simulink model "PF_Simulink_TEST"  (R2022b)
settings: Solver=FixedStepAuto  StartTime=0.0  StopTime=25  FixedStep=0.10  RelTol=1e-3
values from neighbouring files (symbols this model uses):
  D1 = W2_newnew(x0)    [main_S_F.m]
  D2 = W3_newnew(x0)    [main_S_F.m]
  num_particles = 75    [main_S_F.m]
  std_dev1 = std_dev    [main_S_F.m]
  std_dev2 = [1.5; 1.5; 1e-3; 1e-3; 1e-6; 0.2;0.2]    [main_S_F.m]
  W_xu_ranges = [ ... (first row only)    [main_S_F.m]
  W_xucar1 = [10;10;1e-4;1e-4;1e-4;0.50;0.1]    [main_S_F.m]
  W_xucar2 = [10;10;1e-4;1e-4;1e-4;0.50;0.1]    [main_S_F.m]
  x0 = [0;-45;pi/2;0;0;-30;0;0;10;0]    [main_S_F.m]
undefined symbols (not defined in the file or in its folder): estimated_W_xu_car2, estimated_Wxu_car1
(part 1 of 2)
settings Model: PauseTimes=10  Creator=user  LastModifiedBy=user

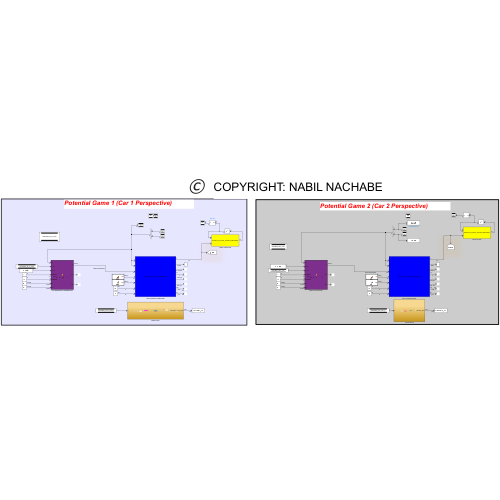
[thumbnail: Simulink's stored preview of the top-level diagram]
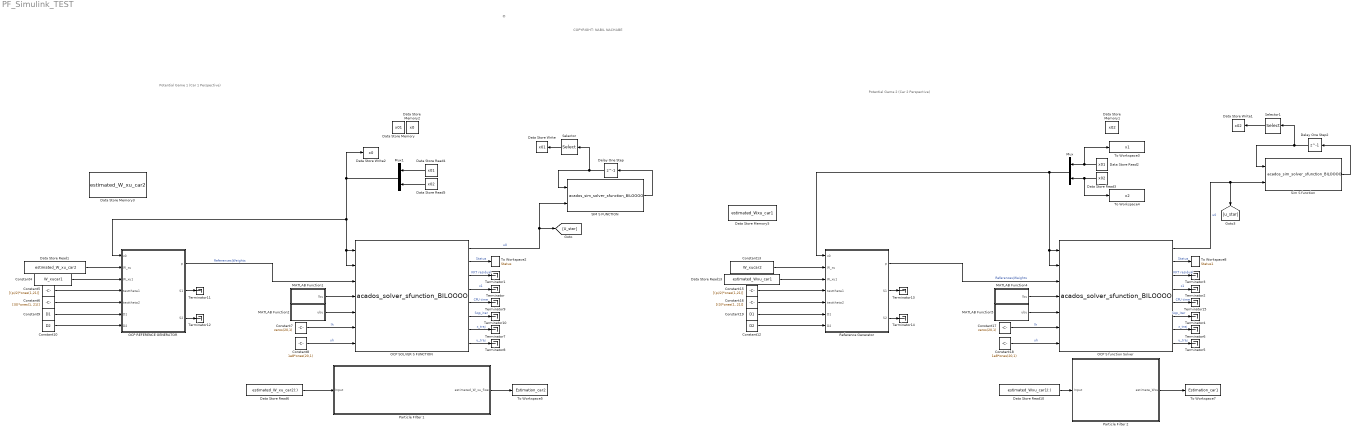
== system PF_Simulink_TEST ==
  note: ©
  note: COPYRIGHT: NABIL NACHABE
  note: Potential Game 2 (Car 2 Perspective)
  note: Potential Game 1 (Car 1 Perspective)
  Constant10 : Constant  Value=D2
  Constant12 : Constant  Value=D2
  Constant13 : Constant  Value=W_xucar2
  Constant15 : Constant  Value=[(pi/2)*ones(1,21)]
  Constant16 : Constant  Value=[(0)*ones(1, 21)]
  Constant17 : Constant  Value=zeros(20,1)
  Constant18 : Constant  Value=1e8*ones(20,1)
  Constant19 : Constant  Value=D1
  Constant4 : Constant  Value=W_xucar1
  Constant5 : Constant  Value=[(pi/2)*ones(1,21)]
  Constant6 : Constant  Value=[(0)*ones(1, 21)]
  Constant7 : Constant  Value=zeros(20,1)
  Constant8 : Constant  Value=1e8*ones(20,1)
  Constant9 : Constant  Value=D1
  Data Store Memory : DataStoreMemory  DataStoreName=x01  WriteAfterWriteMsg=warning  InitialValue=x01  ShowAdditionalParam=off
  Data Store Memory1 : DataStoreMemory  DataStoreName=x02  WriteAfterWriteMsg=warning  InitialValue=x02  ShowAdditionalParam=off
  Data Store Memory2 : DataStoreMemory  DataStoreName=x0  WriteAfterWriteMsg=warning  InitialValue=x0  ShareAcrossModelInstances=on  ShowAdditionalParam=off
  Data Store Memory3 : DataStoreMemory  DataStoreName=estimated_W_xu_car2  WriteAfterWriteMsg=warning  InitialValue=initial_guess_belief_car2  ShowAdditionalParam=off
  Data Store Memory5 : DataStoreMemory  DataStoreName=estimated_Wxu_car1  WriteAfterWriteMsg=warning  InitialValue=initial_guess_belief_car1  ShowAdditionalParam=off
  Data Store Read1 : DataStoreRead  DataStoreName=estimated_W_xu_car2  IndexOptions=Index vector (dialog)  Indices=1  OutputSizes=1
  Data Store Read10 : DataStoreRead  DataStoreName=estimated_Wxu_car1  DataStoreElements=estimated_Wxu_car1(:)  IndexOptions=Index vector (dialog)  Indices=1  OutputSizes=1
  Data Store Read13 : DataStoreRead  DataStoreName=estimated_Wxu_car1  IndexOptions=Index vector (dialog)  Indices=1  OutputSizes=1
  Data Store Read2 : DataStoreRead  DataStoreName=x01  IndexOptions=Index vector (dialog)  Indices=1  OutputSizes=1
  Data Store Read3 : DataStoreRead  DataStoreName=x02  IndexOptions=Index vector (dialog)  Indices=1  OutputSizes=1
  Data Store Read4 : DataStoreRead  DataStoreName=x01  IndexOptions=Index vector (dialog)  Indices=1  OutputSizes=1
  Data Store Read5 : DataStoreRead  DataStoreName=x02  IndexOptions=Index vector (dialog)  Indices=1  OutputSizes=1
  Data Store Read6 : DataStoreRead  DataStoreName=estimated_W_xu_car2  DataStoreElements=estimated_W_xu_car2(:)  IndexOptions=Index vector (dialog)  Indices=1  OutputSizes=1
  Data Store Write : DataStoreWrite  DataStoreName=x01  DataStoreElements=x01  IndexOptions=Index vector (dialog)  Indices=1  OutputSizes=1
  Data Store Write1 : DataStoreWrite  DataStoreName=x02  IndexOptions=Index vector (dialog)  Indices=1  OutputSizes=1
  Data Store Write2 : DataStoreWrite  DataStoreName=x0  IndexOptions=Index vector (dialog)  Indices=1  OutputSizes=1
  Delay One Step : Delay  DelayLength=1  InitialCondition=x0
  Delay One Step2 : Delay  DelayLength=1  InitialCondition=x0
  MATLAB Function1 : MATLAB Function  TreatAsAtomicUnit=on
  MATLAB Function2 : MATLAB Function  TreatAsAtomicUnit=on
  MATLAB Function4 : MATLAB Function  TreatAsAtomicUnit=on
  MATLAB Function5 : MATLAB Function  TreatAsAtomicUnit=on
  Mux : Mux  Inputs=2
  Mux1 : Mux  Inputs=2
  OCP REFERENCE GENERATOR : MATLAB Function  TreatAsAtomicUnit=on
  OCP S function Solver : S-Function  FunctionName=acados_solver_sfunction_BILOOOO  SFunctionDeploymentMode=off  EnableBusSupport=off
  OCP SOLVER S FUNCTION : S-Function  FunctionName=acados_solver_sfunction_BILOOOO  SFunctionDeploymentMode=off  EnableBusSupport=off
  Particle FIlter 1 : Subsystem
  Particle Filter 2 : Subsystem
  Reference Generator : MATLAB Function  TreatAsAtomicUnit=on
  SIM S FUNCTION : S-Function  FunctionName=acados_sim_solver_sfunction_BILOOOO  SFunctionDeploymentMode=off  EnableBusSupport=off
  Selector : Selector  InputPortWidth=10  IndexOptions=Index vector (dialog)  Indices=[1:5]  OutputSizes=1
  Selector1 : Selector  InputPortWidth=10  IndexOptions=Index vector (dialog)  Indices=[6:10]  OutputSizes=1
  Sim S function : S-Function  FunctionName=acados_sim_solver_sfunction_BILOOOO  SFunctionDeploymentMode=off  EnableBusSupport=off
  Terminator{,1..15} (16 alike) : Terminator
  To Workspace2 : ToWorkspace  VariableName=Status  SampleTime=-1
      settings: Save2DSignal=2-D array (concatenate along first dimension)
  To Workspace3 : ToWorkspace  VariableName=x1  SaveFormat=Structure  SampleTime=-1
  To Workspace4 : ToWorkspace  VariableName=x2  SaveFormat=Structure  SampleTime=-1
  To Workspace5 : ToWorkspace  VariableName=Estimation_car2  SampleTime=-1
      settings: Save2DSignal=2-D array (concatenate along first dimension)
  To Workspace7 : ToWorkspace  VariableName=Estimation_car1  SampleTime=-1
      settings: Save2DSignal=2-D array (concatenate along first dimension)
  To Workspace8 : ToWorkspace  VariableName=Status1  SampleTime=-1
      settings: Save2DSignal=2-D array (concatenate along first dimension)
  wires:
  Data Store Read13/1 -> Reference Generator/3(W_xu1)
  Mux1/1 -> Data Store Write2/1, OCP SOLVER S FUNCTION/2, OCP SOLVER S FUNCTION/1, OCP REFERENCE GENERATOR/1(x0)
  Data Store Read5/1 -> Mux1/2
  Sim S function/1 -> Delay One Step2/1
  Constant19/1 -> Reference Generator/6(D1)
  Constant15/1 -> Reference Generator/4(testtheta1)
  Constant7/1 -> OCP SOLVER S FUNCTION/6  "lh"
  MATLAB Function1/1(lbu) -> OCP SOLVER S FUNCTION/4
  OCP REFERENCE GENERATOR/2(S1) -> Terminator11/1
  OCP REFERENCE GENERATOR/1(p) -> OCP SOLVER S FUNCTION/3  "References|Weights"
  OCP SOLVER S FUNCTION/4 -> Terminator/1  "x1"
  Data Store Read3/1 -> To Workspace4/1, Mux/2
  Reference Generator/3(S2) -> Terminator14/1
  OCP S function Solver/7 -> Terminator6/1  "x_traj"
  OCP SOLVER S FUNCTION/3 -> Terminator1/1  "KKT residual"
  MATLAB Function4/1(lbu) -> OCP S function Solver/4
  Delay One Step/1 -> Selector/1, SIM S FUNCTION/1
  Constant13/1 -> Reference Generator/2(W_xu)
  Constant17/1 -> OCP S function Solver/6  "lh"
  SIM S FUNCTION/1 -> Delay One Step/1
  Constant8/1 -> OCP SOLVER S FUNCTION/7  "uh"
  OCP REFERENCE GENERATOR/3(S2) -> Terminator12/1
  Delay One Step2/1 -> Selector1/1, Sim S function/1
  OCP SOLVER S FUNCTION/2 -> To Workspace2/1  "Status"
  OCP S function Solver/2 -> To Workspace8/1  "Status"
  Reference Generator/1(p) -> OCP S function Solver/3  "References|Weights"
  MATLAB Function5/1(ubu) -> OCP S function Solver/5
  OCP S function Solver/3 -> Terminator3/1  "KKT residual"
  Constant10/1 -> OCP REFERENCE GENERATOR/7(D2)
  OCP SOLVER S FUNCTION/8 -> Terminator8/1  "u_traj"
  OCP S function Solver/5 -> Terminator15/1  "CPU time"
  OCP S function Solver/4 -> Terminator2/1  "x1"
  Constant4/1 -> OCP REFERENCE GENERATOR/3(W_xu1)
  Constant16/1 -> Reference Generator/5(testtheta2)
  MATLAB Function2/1(ubu) -> OCP SOLVER S FUNCTION/5
  Mux/1 -> OCP S function Solver/2, OCP S function Solver/1, Reference Generator/1(x0)
  Data Store Read4/1 -> Mux1/1
  OCP S function Solver/6 -> Terminator4/1  "Sqp_iter"
  Constant6/1 -> OCP REFERENCE GENERATOR/5(testtheta2)
  OCP S function Solver/1 -> Sim S function/2, [u_star]  "u0"
  OCP SOLVER S FUNCTION/6 -> Terminator10/1  "Sqp_iter"
  OCP SOLVER S FUNCTION/1 -> SIM S FUNCTION/2, [U_star]  "u0"
  Reference Generator/2(S1) -> Terminator13/1
  OCP S function Solver/8 -> Terminator5/1  "u_traj"
  Constant5/1 -> OCP REFERENCE GENERATOR/4(testtheta1)
  Selector/1 -> Data Store Write/1
  Selector1/1 -> Data Store Write1/1
  OCP SOLVER S FUNCTION/5 -> Terminator9/1  "CPU time"
  Constant9/1 -> OCP REFERENCE GENERATOR/6(D1)
  OCP SOLVER S FUNCTION/7 -> Terminator7/1  "x_traj"
  Data Store Read2/1 -> To Workspace3/1, Mux/1
  Constant12/1 -> Reference Generator/7(D2)
  Constant18/1 -> OCP S function Solver/7  "uh"
  Data Store Read1/1 -> OCP REFERENCE GENERATOR/2(W_xu)
  Data Store Read6/1 -> Particle FIlter 1/1(Input)
  Particle FIlter 1/1(estimated_W_xu_fixed) -> To Workspace5/1
  Data Store Read10/1 -> Particle Filter 2/1(Input)
  Particle Filter 2/1(estimate_Wxu) -> To Workspace7/1

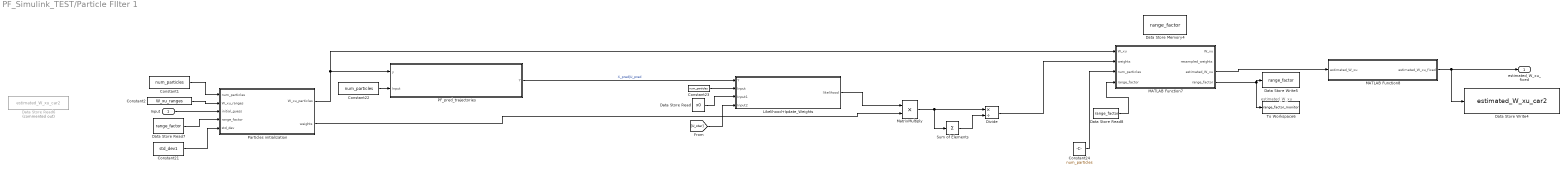
== system PF_Simulink_TEST/Particle FIlter 1 ==
  note: estimated_W_xu
  Input : Inport
  Constant{1,22..24} (4 alike) : Constant  Value=num_particles
  Constant2 : Constant  Value=W_xu_ranges
  Constant21 : Constant  Value=std_dev1
  Data Store Memory4 : DataStoreMemory  DataStoreName=range_factor  WriteAfterWriteMsg=warning  InitialValue=1  ShowAdditionalParam=off
  Data Store Read : DataStoreRead  DataStoreName=x0  IndexOptions=Index vector (dialog)  Indices=1  OutputSizes=1
  Data Store Read6 : DataStoreRead  Commented=on  DataStoreName=estimated_W_xu_car2  IndexOptions=Index vector (dialog)  Indices=1  OutputSizes=1
  Data Store Read7 : DataStoreRead  DataStoreName=range_factor  IndexOptions=Index vector (dialog)  Indices=1  OutputSizes=1
  Data Store Read8 : DataStoreRead  DataStoreName=range_factor  IndexOptions=Index vector (dialog)  Indices=1  OutputSizes=1
  Data Store Write4 : DataStoreWrite  DataStoreName=estimated_W_xu_car2  IndexOptions=Index vector (dialog)  Indices=1  OutputSizes=1
  Data Store Write5 : DataStoreWrite  DataStoreName=range_factor  IndexOptions=Index vector (dialog)  Indices=1  OutputSizes=1
  Divide : Product  Inputs=*/
  Likelihood+Ipdate_Weights : Subsystem  TreatAsAtomicUnit=on
  MATLAB Function7 : MATLAB Function  TreatAsAtomicUnit=on
  MATLAB Function8 : MATLAB Function  TreatAsAtomicUnit=on
  MatrixMultiply : Product
  PF_pred_trajectories : Subsystem  TreatAsAtomicUnit=on
  Particles initialization : MATLAB Function  TreatAsAtomicUnit=on
  Sum of Elements : Sum  Inputs=+
  To Workspace6 : ToWorkspace  VariableName=range_factor_monitor  SampleTime=-1
      settings: Save2DSignal=2-D array (concatenate along first dimension)
  estimated_W_xu_fixed : Outport
  wires:
  Data Store Read7/1 -> Particles initialization/4(range_factor)
  Constant1/1 -> Particles initialization/1(num_particles)
  MATLAB Function8/1(estimated_W_xu_fixed) -> Data Store Write4/1, estimated_W_xu_fixed/1
  Constant23/1 -> Likelihood+Ipdate_Weights/2(Input)
  Particles initialization/1(W_xu_particles) -> MATLAB Function7/1("W_xu "), PF_pred_trajectories/1(y)
  Constant22/1 -> PF_pred_trajectories/2(Input)
  PF_pred_trajectories/1(Y) -> Likelihood+Ipdate_Weights/1(Y)  "X_pred|U_pred"
  Likelihood+Ipdate_Weights/1(likelihood) -> MatrixMultiply/1
  Sum of Elements/1 -> Divide/2
  Particles initialization/2(weights) -> MatrixMultiply/2
  Data Store Read/1 -> Likelihood+Ipdate_Weights/3(Input1)
  Constant24/1 -> MATLAB Function7/3(num_particles)
  MatrixMultiply/1 -> Sum of Elements/1, Divide/1
  Data Store Read8/1 -> MATLAB Function7/4("range_factor ")
  MATLAB Function7/4(range_factor) -> Data Store Write5/1, To Workspace6/1
  MATLAB Function7/3(estimated_W_xu) -> MATLAB Function8/1(estimated_W_xu)
  [U_star] -> Likelihood+Ipdate_Weights/4(Input2)
  Constant2/1 -> Particles initialization/2(W_xu_ranges)
  Divide/1 -> MATLAB Function7/2(weights)
  Input/1 -> Particles initialization/3(initial_guess)
  Constant21/1 -> Particles initialization/5(std_dev)

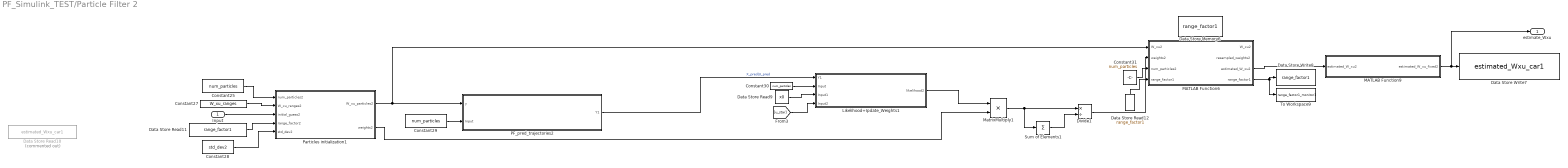
== system PF_Simulink_TEST/Particle Filter 2 ==
  Input : Inport
  Constant{25,29..31} (4 alike) : Constant  Value=num_particles
  Constant27 : Constant  Value=W_xu_ranges
  Constant28 : Constant  Value=std_dev2
  Data Store Memory6 : DataStoreMemory  DataStoreName=range_factor1  WriteAfterWriteMsg=warning  InitialValue=1  ShowAdditionalParam=off
  Data Store Read10 : DataStoreRead  Commented=on  DataStoreName=estimated_Wxu_car1  IndexOptions=Index vector (dialog)  Indices=1  OutputSizes=1
  Data Store Read11 : DataStoreRead  DataStoreName=range_factor1  IndexOptions=Index vector (dialog)  Indices=1  OutputSizes=1
  Data Store Read12 : DataStoreRead  DataStoreName=range_factor1  IndexOptions=Index vector (dialog)  Indices=1  OutputSizes=1
  Data Store Read9 : DataStoreRead  DataStoreName=x0  IndexOptions=Index vector (dialog)  Indices=1  OutputSizes=1
  Data Store Write7 : DataStoreWrite  DataStoreName=estimated_Wxu_car1  IndexOptions=Index vector (dialog)  Indices=1  OutputSizes=1
  Data Store Write8 : DataStoreWrite  DataStoreName=range_factor1  IndexOptions=Index vector (dialog)  Indices=1  OutputSizes=1
  Divide1 : Product  Inputs=*/
  Likelihood+Ipdate_Weights1 : Subsystem  TreatAsAtomicUnit=on
  MATLAB Function6 : MATLAB Function  TreatAsAtomicUnit=on
  MATLAB Function9 : MATLAB Function  TreatAsAtomicUnit=on
  MatrixMultiply1 : Product
  PF_pred_trajectories2 : Subsystem  TreatAsAtomicUnit=on
  Particles initialization1 : MATLAB Function  TreatAsAtomicUnit=on
  Sum of Elements1 : Sum  Inputs=+
  To Workspace9 : ToWorkspace  VariableName=range_factor1_monitor1  SampleTime=-1
      settings: Save2DSignal=2-D array (concatenate along first dimension)
  estimate_Wxu : Outport
  wires:
  Particles initialization1/1(W_xu_particles2) -> MATLAB Function6/1("W_xu2 "), PF_pred_trajectories2/1(y)
  Likelihood+Ipdate_Weights1/1(likelihood2) -> MatrixMultiply1/1
  MATLAB Function6/3(estimated_W_xu2) -> MATLAB Function9/1(estimated_W_xu2)
  Data Store Read12/1 -> MATLAB Function6/4("range_factor1 ")
  MATLAB Function9/1(estimated_W_xu_fixed2) -> estimate_Wxu/1, Data Store Write7/1
  Constant31/1 -> MATLAB Function6/3(num_particles2)
  Constant27/1 -> Particles initialization1/2(W_xu_ranges2)
  Data Store Read9/1 -> Likelihood+Ipdate_Weights1/3(Input1)
  Divide1/1 -> MATLAB Function6/2(weights2)
  MATLAB Function6/4(range_factor1) -> Data Store Write8/1, To Workspace9/1
  Constant29/1 -> PF_pred_trajectories2/2(Input)
  MatrixMultiply1/1 -> Divide1/1, Sum of Elements1/1
  Data Store Read11/1 -> Particles initialization1/4(range_factor2)
  Constant30/1 -> Likelihood+Ipdate_Weights1/2(Input)
  Particles initialization1/2(weights2) -> MatrixMultiply1/2
  [u_star] -> Likelihood+Ipdate_Weights1/4(Input2)
  Constant25/1 -> Particles initialization1/1(num_particles2)
  Constant28/1 -> Particles initialization1/5(std_dev2)
  Sum of Elements1/1 -> Divide1/2
  PF_pred_trajectories2/1(Y1) -> Likelihood+Ipdate_Weights1/1(Y1)  "X_pred|U_pred"
  Input/1 -> Particles initialization1/3(initial_guess2)

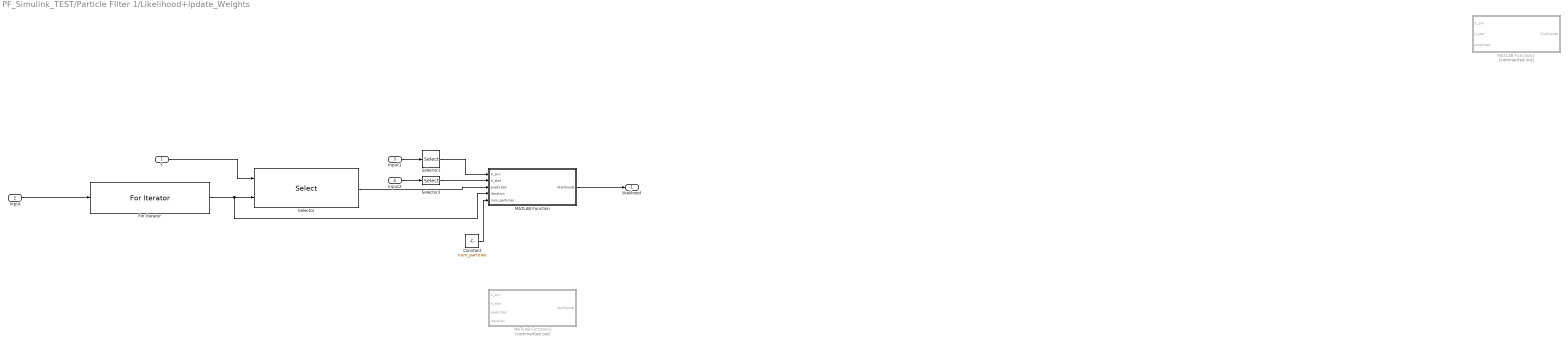
== system PF_Simulink_TEST/Particle FIlter 1/Likelihood+Ipdate_Weights ==
  Y : Inport
  Input : Inport  Port=2
  Input1 : Inport  Port=3
  Input2 : Inport  Port=4
  Constant : Constant  Value=num_particles
  For Iterator : ForIterator  IterationSource=external
  MATLAB Function : MATLAB Function  TreatAsAtomicUnit=on
  MATLAB Function1 : MATLAB Function  Commented=on  TreatAsAtomicUnit=on
  MATLAB Function2 : MATLAB Function  Commented=on  TreatAsAtomicUnit=on
  Selector : Selector  NumberOfDimensions=2  IndexOptions=Select all,Index vector (port)  Indices=[1 3],1  OutputSizes=1,1  RuntimeRangeChecks=on
  Selector1 : Selector  InputPortWidth=10  IndexOptions=Index vector (dialog)  Indices=[6:10]  OutputSizes=1
  Selector2 : Selector  InputPortWidth=4  IndexOptions=Index vector (dialog)  Indices=[3:4]  OutputSizes=1
  likelihood : Outport
  wires:
  Input/1 -> For Iterator/1
  For Iterator/1 -> MATLAB Function/4(iteration), Selector/2
  Y/1 -> Selector/1
  MATLAB Function/1(likelihoods) -> likelihood/1
  Constant/1 -> MATLAB Function/5(num_particles)
  Input1/1 -> Selector1/1
  Selector1/1 -> MATLAB Function/1(X_sim)
  Input2/1 -> Selector2/1
  Selector2/1 -> MATLAB Function/2(U_star)
  Selector/1 -> MATLAB Function/3(predicted)

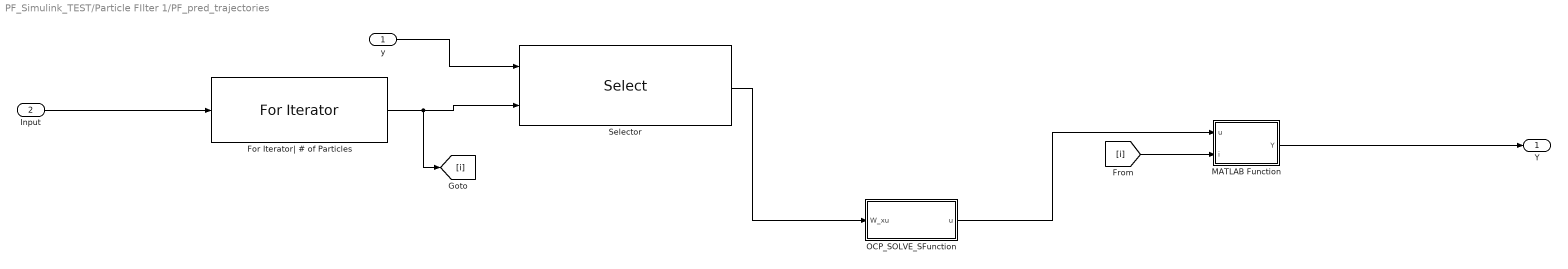
== system PF_Simulink_TEST/Particle FIlter 1/PF_pred_trajectories ==
  y : Inport
  Input : Inport  Port=2
  For Iterator| # of Particles : ForIterator  IterationSource=external  IterationLimit=num_particles
  MATLAB Function : MATLAB Function  TreatAsAtomicUnit=on
  OCP_SOLVE_SFunction : Subsystem
  Selector : Selector  NumberOfDimensions=2  IndexOptions=Index vector (port),Select all  Indices=[1 3],1  OutputSizes=1,1  RuntimeRangeChecks=on
  Y : Outport
  wires:
  Input/1 -> For Iterator| # of Particles/1
  For Iterator| # of Particles/1 -> [i], Selector/2
  y/1 -> Selector/1
  Selector/1 -> OCP_SOLVE_SFunction/1(W_xu)
  OCP_SOLVE_SFunction/1(u) -> MATLAB Function/1(u)
  [i] -> MATLAB Function/2(i)
  MATLAB Function/1(Y) -> Y/1

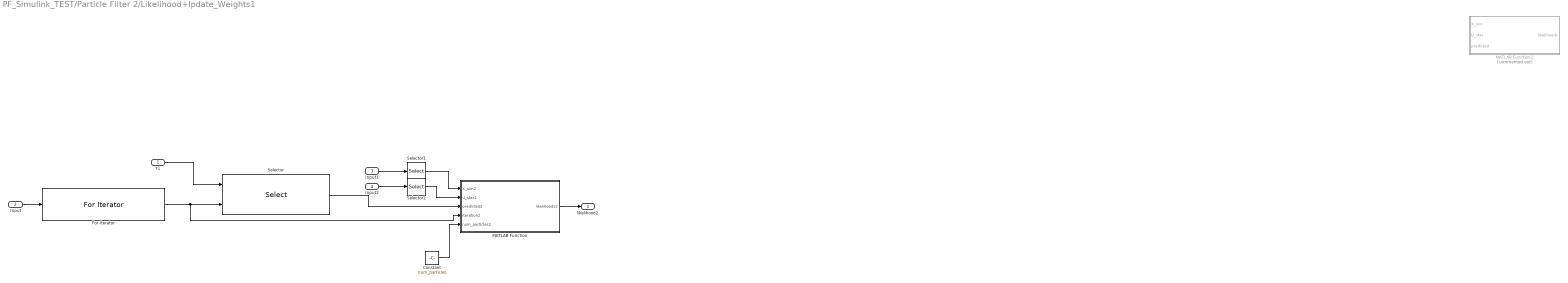
== system PF_Simulink_TEST/Particle Filter 2/Likelihood+Ipdate_Weights1 ==
  Y1 : Inport
  Input : Inport  Port=2
  Input1 : Inport  Port=3
  Input2 : Inport  Port=4
  Constant : Constant  Value=num_particles
  For Iterator : ForIterator  IterationSource=external
  MATLAB Function : MATLAB Function  TreatAsAtomicUnit=on
  MATLAB Function1 : MATLAB Function  Commented=on  TreatAsAtomicUnit=on
  Selector : Selector  NumberOfDimensions=2  IndexOptions=Select all,Index vector (port)  Indices=[1 3],1  OutputSizes=1,1  RuntimeRangeChecks=on
  Selector1 : Selector  InputPortWidth=10  IndexOptions=Index vector (dialog)  Indices=[1:5]  OutputSizes=1
  Selector2 : Selector  InputPortWidth=4  IndexOptions=Index vector (dialog)  Indices=[1:2]  OutputSizes=1
  likelihood2 : Outport
  wires:
  Constant/1 -> MATLAB Function/5(num_particles2)
  MATLAB Function/1(likelihoods2) -> likelihood2/1
  Selector/1 -> MATLAB Function/3(predicted2)
  Y1/1 -> Selector/1
  For Iterator/1 -> Selector/2, MATLAB Function/4(iteration2)
  Input/1 -> For Iterator/1
  Input1/1 -> Selector1/1
  Selector1/1 -> MATLAB Function/1(X_sim2)
  Input2/1 -> Selector2/1
  Selector2/1 -> MATLAB Function/2(U_star2)

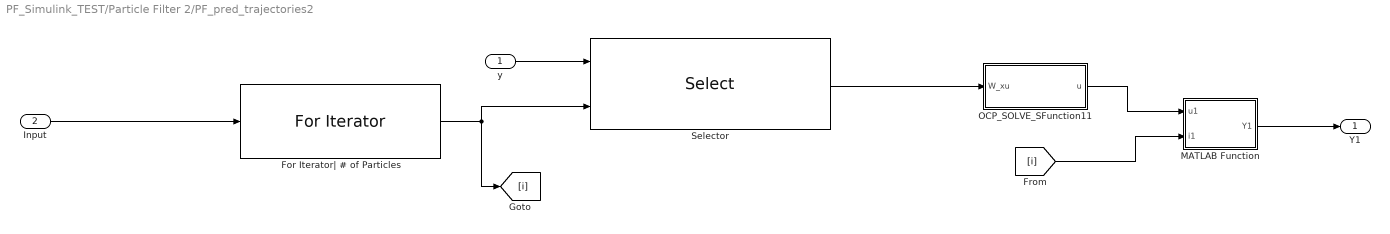
== system PF_Simulink_TEST/Particle Filter 2/PF_pred_trajectories2 ==
  y : Inport
  Input : Inport  Port=2
  For Iterator| # of Particles : ForIterator  IterationSource=external  IterationLimit=num_particles
  MATLAB Function : MATLAB Function  TreatAsAtomicUnit=on
  OCP_SOLVE_SFunction11 : Subsystem
  Selector : Selector  NumberOfDimensions=2  IndexOptions=Index vector (port),Select all  Indices=[1 3],1  OutputSizes=1,1  RuntimeRangeChecks=on
  Y1 : Outport
  wires:
  MATLAB Function/1(Y1) -> Y1/1
  [i] -> MATLAB Function/2(i1)
  OCP_SOLVE_SFunction11/1(u) -> MATLAB Function/1(u1)
  Selector/1 -> OCP_SOLVE_SFunction11/1(W_xu)
  y/1 -> Selector/1
  For Iterator| # of Particles/1 -> Selector/2, [i]
  Input/1 -> For Iterator| # of Particles/1

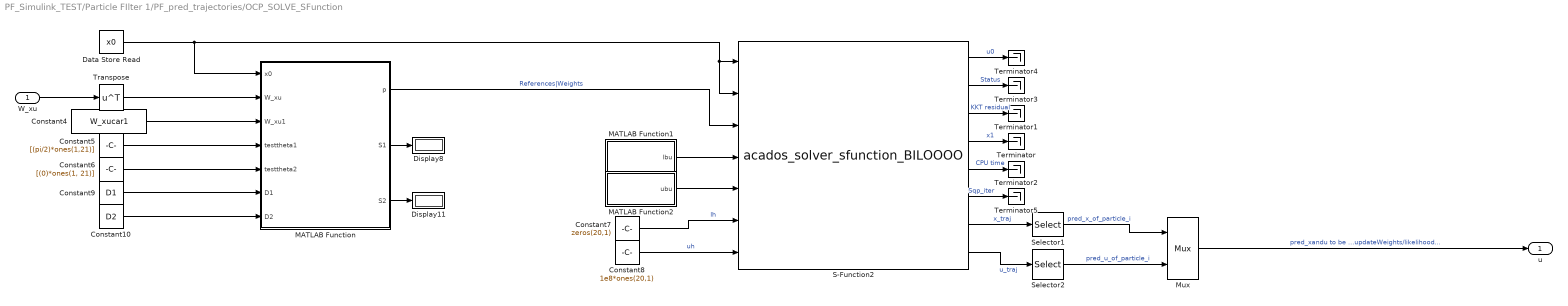
== system PF_Simulink_TEST/Particle FIlter 1/PF_pred_trajectories/OCP_SOLVE_SFunction ==
  W_xu : Inport
  Constant10 : Constant  Value=D2
  Constant4 : Constant  Value=W_xucar1
  Constant5 : Constant  Value=[(pi/2)*ones(1,21)]
  Constant6 : Constant  Value=[(0)*ones(1, 21)]
  Constant7 : Constant  Value=zeros(20,1)
  Constant8 : Constant  Value=1e8*ones(20,1)
  Constant9 : Constant  Value=D1
  Data Store Read : DataStoreRead  DataStoreName=x0  IndexOptions=Index vector (dialog)  Indices=1  OutputSizes=1
  Display11 : Display
  Display8 : Display
  MATLAB Function : MATLAB Function  TreatAsAtomicUnit=on
  MATLAB Function1 : MATLAB Function  TreatAsAtomicUnit=on
  MATLAB Function2 : MATLAB Function  TreatAsAtomicUnit=on
  Mux : Mux  Inputs=2
  S-Function2 : S-Function  FunctionName=acados_solver_sfunction_BILOOOO  SFunctionDeploymentMode=off  EnableBusSupport=off
  Selector1 : Selector  InputPortWidth=210  IndexOptions=Index vector (dialog)  Indices=[11:20]  OutputSizes=1
  Selector2 : Selector  InputPortWidth=80  IndexOptions=Index vector (dialog)  Indices=[1:4]  OutputSizes=1
  Terminator{,1..5} (6 alike) : Terminator
  Transpose : Math  Operator=transpose
  u : Outport
  wires:
  MATLAB Function1/1(lbu) -> S-Function2/4
  Data Store Read/1 -> S-Function2/2, S-Function2/1, MATLAB Function/1(x0)
  S-Function2/3 -> Terminator1/1  "KKT residual"
  Constant6/1 -> MATLAB Function/5(testtheta2)
  MATLAB Function/2(S1) -> Display8/1
  S-Function2/7 -> Selector1/1  "x_traj"
  Constant4/1 -> MATLAB Function/3(W_xu1)
  MATLAB Function/1(p) -> S-Function2/3  "References|Weights"
  S-Function2/6 -> Terminator5/1  "Sqp_iter"
  MATLAB Function2/1(ubu) -> S-Function2/5
  Constant8/1 -> S-Function2/7  "uh"
  S-Function2/5 -> Terminator2/1  "CPU time"
  Constant5/1 -> MATLAB Function/4(testtheta1)
  MATLAB Function/3(S2) -> Display11/1
  Constant9/1 -> MATLAB Function/6(D1)
  S-Function2/4 -> Terminator/1  "x1"
  S-Function2/2 -> Terminator3/1  "Status"
  Constant10/1 -> MATLAB Function/7(D2)
  S-Function2/8 -> Selector2/1  "u_traj"
  Constant7/1 -> S-Function2/6  "lh"
  S-Function2/1 -> Terminator4/1  "u0"
  Selector1/1 -> Mux/1  "pred_x_of_particle_i"
  Selector2/1 -> Mux/2  "pred_u_of_particle_i"
  Mux/1 -> u/1  "pred_xandu to be fed into the updateWeights/likelihood..."
  W_xu/1 -> Transpose/1
  Transpose/1 -> MATLAB Function/2(W_xu)

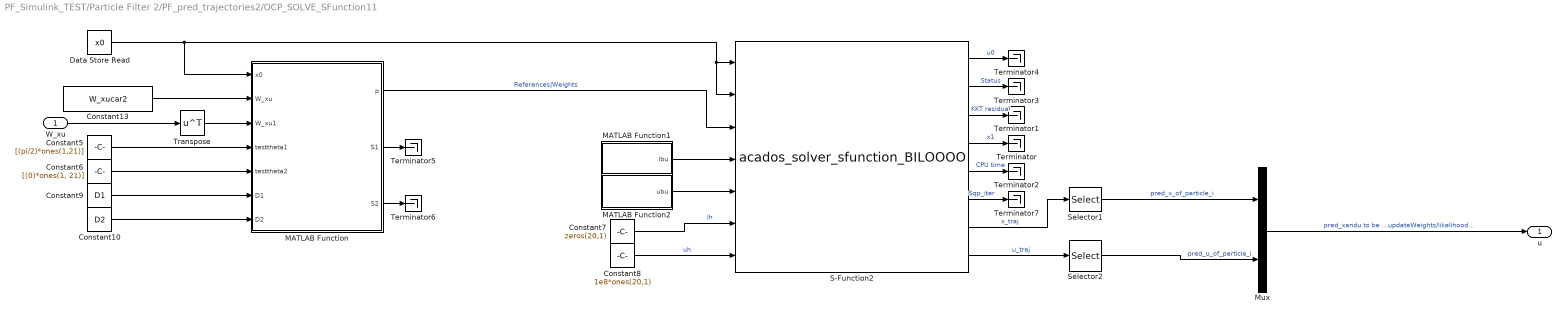
== system PF_Simulink_TEST/Particle Filter 2/PF_pred_trajectories2/OCP_SOLVE_SFunction11 ==
  W_xu : Inport
  Constant10 : Constant  Value=D2
  Constant13 : Constant  Value=W_xucar2
  Constant5 : Constant  Value=[(pi/2)*ones(1,21)]
  Constant6 : Constant  Value=[(0)*ones(1, 21)]
  Constant7 : Constant  Value=zeros(20,1)
  Constant8 : Constant  Value=1e8*ones(20,1)
  Constant9 : Constant  Value=D1
  Data Store Read : DataStoreRead  DataStoreName=x0  IndexOptions=Index vector (dialog)  Indices=1  OutputSizes=1
  MATLAB Function : MATLAB Function  TreatAsAtomicUnit=on
  MATLAB Function1 : MATLAB Function  TreatAsAtomicUnit=on
  MATLAB Function2 : MATLAB Function  TreatAsAtomicUnit=on
  Mux : Mux  Inputs=2
  S-Function2 : S-Function  FunctionName=acados_solver_sfunction_BILOOOO  SFunctionDeploymentMode=off  EnableBusSupport=off
  Selector1 : Selector  InputPortWidth=210  IndexOptions=Index vector (dialog)  Indices=[11:20]  OutputSizes=1
  Selector2 : Selector  InputPortWidth=80  IndexOptions=Index vector (dialog)  Indices=[1:4]  OutputSizes=1
  Terminator{,1..7} (8 alike) : Terminator
  Transpose : Math  Operator=transpose
  u : Outport
  wires:
  W_xu/1 -> Transpose/1
  Mux/1 -> u/1  "pred_xandu to be fed into the updateWeights/likelihood..."
  Selector2/1 -> Mux/2  "pred_u_of_particle_i"
  Selector1/1 -> Mux/1  "pred_x_of_particle_i"
  S-Function2/1 -> Terminator4/1  "u0"
  Constant7/1 -> S-Function2/6  "lh"
  S-Function2/8 -> Selector2/1  "u_traj"
  Constant10/1 -> MATLAB Function/7(D2)
  S-Function2/2 -> Terminator3/1  "Status"
  S-Function2/4 -> Terminator/1  "x1"
  Constant9/1 -> MATLAB Function/6(D1)
  MATLAB Function/3(S2) -> Terminator6/1
  Constant5/1 -> MATLAB Function/4(testtheta1)
  S-Function2/5 -> Terminator2/1  "CPU time"
  Constant8/1 -> S-Function2/7  "uh"
  MATLAB Function2/1(ubu) -> S-Function2/5
  S-Function2/6 -> Terminator7/1  "Sqp_iter"
  MATLAB Function/1(p) -> S-Function2/3  "References|Weights"
  S-Function2/7 -> Selector1/1  "x_traj"
  MATLAB Function/2(S1) -> Terminator5/1
  Constant6/1 -> MATLAB Function/5(testtheta2)
  S-Function2/3 -> Terminator1/1  "KKT residual"
  Data Store Read/1 -> MATLAB Function/1(x0), S-Function2/1, S-Function2/2
  MATLAB Function1/1(lbu) -> S-Function2/4
  Constant13/1 -> MATLAB Function/2(W_xu)
  Transpose/1 -> MATLAB Function/3(W_xu1)

== matlab function PF_Simulink_TEST/Particle FIlter 1/Particles initialization ==
  data: num_particles input; W_xu_particles output size=[num_particles, 7] [..100000]; W_xu_ranges input; initial_guess input; range_factor input; std_dev input; weights output size=[num_particles,1] [-1..10]
function [W_xu_particles,weights] = initializeParticles1(num_particles, W_xu_ranges,initial_guess,range_factor,std_dev)
    num_ranges = size(W_xu_ranges, 1);  % Number of parameters
    W_xu_particles = zeros(num_particles, num_ranges);

    std_dev=std_dev*range_factor;

    
    for i = 1:num_ranges
        % Define the mean and standard deviation for the Gaussian distribution for parameter i
        mean_value = initial_guess(i);  % Mean for the Gaussian distribution
        std_deviation = std_dev(i);          % Standard deviation for the Gaussian distribution

        % Generate random particles from a Gaussian distribution
        W_xu_particles(:, i) = mean_value + std_deviation * randn(num_particles, 1);
        
        % Clip values to be within the specified range
        W_xu_particles(:, i) = max(W_xu_ranges(i, 1), min(W_xu_ranges(i, 2), W_xu_particles(:, i)));
    end
    %%% make the x and y the same since we have that knowledge (testing this)
    W_xu_particles(:,2)=W_xu_particles(:,1);
    %%%
    
    % Initialize weights uniformly
    weights = ones(num_particles, 1) / num_particles;
%     
%     particles.W_xu = W_xu_particles;
%     particles.weights = weights;
end

== matlab function PF_Simulink_TEST/Particle FIlter 1/Likelihood+Ipdate_Weights/MATLAB Function ==
  data: X_sim input; U_star input; likelihoods output size=[num_particles,1]; predicted input; iteration input; num_particles input
function likelihoods = computeLikelihood(X_sim, U_star, predicted, iteration, num_particles)
    % Inputs:
    % X_sim: Actual state trajectory (Nx1)
    % U_star: Actual control inputs (Nu x 1)
    % predicted: A matrix containing both predicted trajectory and control inputs (14 x num_particles)
    % iteration: Current iteration index from the for iterator
    % num_particles: Number of particles used

%     % Initialize likelihood_storage to zeros at the start of each PF
%     persistent likelihood_storage;
% 
%     % Initialize on the first call or reset after each PF
%     if isempty(likelihood_storage) || length(likelihood_storage) ~= num_particles
%         likelihood_storage = zeros(num_particles, 1); % Initialize as zeros
%     end
    likelihood_storage=zeros(num_particles,1);

    % Parameters
    std_state = [0.1; 0.1; 0.01; 0.05; 0.02];  % For (x, y, theta, velocity, steering)
    std_control = [0.1; 0.01];  % For (acceleration, steering rate)

    % Extract predicted trajectory and control inputs for the current particle
%     predicted_trajectory = predicted(1:10); % First 10 elements for states
%     predicted_control = predicted(11:14);   % Last 4 elements for control inputs
    predicted_trajectory = predicted(6:10); % First 10 elements for states
    predicted_control = predicted(13:14);   % Last 4 elements for control inputs

    % Compute the deviation between predicted and observed state trajectory
    state_deviation = X_sim - predicted_trajectory;

    % Compute the deviation between predicted and observed control inputs
    control_deviation = U_star - predicted_control;

    % Compute weighted errors
    weighted_state_error = sum(state_deviation.^2);
    weighted_control_error = sum(control_deviation.^2);

    % Combine state and control errors
    total_error = weighted_state_error + weighted_control_error;
    scaling_factor = 10 / (max(std(state_deviation(:)), std(control_deviation(:))) + 1e-5); % Adjust as necessary

    % Compute likelihood
    likelihood = exp(-0.5 * scaling_factor * total_error);
    likelihood = max(likelihood, 1e-30); % Ensure likelihood is within reasonable range

    % Update the likelihood storage for the current iteration
    likelihood_storage(iteration) = likelihood;

    % Output the accumulated likelihoods
    likelihoods = likelihood_storage; % Output the accumulated likelihoods
end

== matlab function PF_Simulink_TEST/Particle FIlter 1/Likelihood+Ipdate_Weights/MATLAB Function1 ==
  data: X_sim input; U_star input; likelihoods output; predicted input
% function [likelihood, total_error] = computeLikelihood(X_sim, predicted_trajectory, U_star)
%     % Extract state and control inputs
%     nx = 10;  % Number of state variables
%     nu = 4;   % Number of control inputs
% 
%     % Assuming predicted_trajectory is a 14x1 vector
%     predicted_states = predicted_trajectory(1:nx); % First 10 elements for states
%     predicted_control = predicted_trajectory(nx+1:end); % Last 4 elements for controls
% 
%     std_state = [0.1; 0.1; 0.01; 0.05; 0.02];  % For (x, y, theta, velocity, steering)
%     std_control = [0.1; 0.01];  % For (acceleration, steering rate)
% 
%     % Compute the deviation between predicted and observed state trajectory
%     state_deviation = X_sim - predicted_states;
% 
%     % Compute the deviation between predicted and observed control inputs
%     control_deviation = U_star - predicted_control;
% 
%     % Assuming state variables are weighted
%     importance_state_weights = [1, 1, 1e-5, 1e-5, 1e-5]; % Weights for state variables
%     importance_control_weights = [1, 1];                 % Weights for control inputs
%     
%     % Noise-based weights
%     noise_state_weights = 1 ./ (2 * std_state.^2);  % State noise
%     noise_control_weights = 2 * std_control.^2;  % Control noise
% 
%     combined_state_weights = importance_state_weights ./ (1 + noise_state_weights);
%     normalized_weights_state = combined_state_weights / sum(combined_state_weights);
% 
%     combined_control_weights = importance_control_weights .* (1 ./ (1 + noise_control_weights));
%     normalized_weights_control = combined_control_weights / sum(combined_control_weights);
% 
%     % Compute weighted state and control errors
%     weighted_state_error = sum((normalized_weights_state' .* state_deviation).^2, 1);
%     weighted_control_error = sum((normalized_weights_control' .* control_deviation).^2, 1);
% 
%     % Combine state and control errors
%     total_error = sum(weighted_state_error) + sum(weighted_control_error);
% 
%     norm_state_error = state_deviation ./ (std(state_deviation(:)) + 1e-5);
%     norm_control_error = control_deviation ./ (std(control_deviation(:)) + 1e-5);
%     
%     scaling_factor = 10 * 1 / (max(std(norm_state_error), std(norm_control_error)) + 1e-5);
% 
%     % Compute likelihood
%     likelihood = exp(-0.5 * scaling_factor * total_error);
%     likelihood = max(likelihood, 1e-30); % Ensure likelihood is within a reasonable range
% end

function likelihoods = computeLikelihoods(X_sim, U_star, predicted)
    % Inputs:
    % X_sim: Actual state trajectory (Nx1)
    % U_star: Actual control inputs (Nu x 1)
    % predicted: A matrix containing both predicted trajectory and control inputs (14 x num_particles)

    % Parameters
    num_particles = size(predicted, 2); % Number of particles
    likelihoods = zeros(num_particles, 1); % Preallocate array for likelihoods

    std_state = [0.1; 0.1; 0.01; 0.05; 0.02];  % For (x, y, theta, velocity, steering)
    std_control = [0.1; 0.01];  % For (acceleration, steering rate)

    % Loop through each particle
    for i = 1:num_particles
        % Extract predicted trajectory and control inputs for the current particle
        predicted_trajectory = predicted(1:10, i); % First 10 elements for states
        predicted_control = predicted(11:14, i);   % Last 4 elements for control inputs

        % Compute the deviation between predicted and observed state trajectory
        state_deviation = X_sim - predicted_trajectory;

        % Compute the deviation between predicted and observed control inputs
        control_deviation = U_star - predicted_control;

        % Compute weighted errors (adjust according to your weighting scheme)
        weighted_state_error = sum(state_deviation.^2);
        weighted_control_error = sum(control_deviation.^2);

        % Combine state and control errors
        total_error = weighted_state_error + weighted_control_error;
        scaling_factor = 10 / (max(std(state_deviation(:)), std(control_deviation(:))) + 1e-5); % Adjust as necessary

        % Compute likelihood
        likelihood = exp(-0.5 * scaling_factor * total_error);
        likelihood = max(likelihood, 1e-30); % Ensure likelihood is within reasonable range

        % Store the likelihood for this particle
        likelihoods(i) = likelihood;
    end
end

== matlab function PF_Simulink_TEST/Particle FIlter 1/MATLAB Function7 ==
  data: W_xu input; W_xu output; resampled_weights output size=[num_particles,1]; weights input; num_particles input; estimated_W_xu output size=[1,7]; range_factor output; range_factor input
function [W_xu, resampled_weights,estimated_W_xu,range_factor] = resampleParticles(W_xu, weights,num_particles,range_factor)
    % Inputs:
    % - W_xu: Matrix of particle states and weights (num_particles x 7)
    % - weights: Current particle weights (num_particles x 1)
    %
    % Outputs:
    % - W_xu: Resampled particle matrix (num_particles x 7)
    % - resampled_weights: Uniform weights after resampling (num_particles x 1)

  
    % Normalize weights
%     weights = weights / sum(weights);

    % Resample particle indices based on the updated weights
    estimated_W_xu=zeros(1,7);
    resampled_weights=zeros(num_particles,1);

    resample_indices = randsample(1:num_particles, num_particles, true, weights);

    % Resample particles using the indices
    W_xu = W_xu(resample_indices, :); 

    % Reset weights to uniform distribution after resampling
    resampled_weights = ones(num_particles, 1) / num_particles;

    % Return the updated W_xu, pre-resample weights, and resampled weights


     % Element-wise multiplication of W_xu by weights
    weighted_W_xu = W_xu .* resampled_weights;

    % Sum the weighted values across the particles (i.e., summing along rows)
    estimated_W_xu = sum(weighted_W_xu, 1); % Output will be 1x7
    range_factor=range_factor*0.975;
    range_factor=max(0.10,range_factor);
end

== matlab function PF_Simulink_TEST/Particle FIlter 1/MATLAB Function8 ==
  data: estimated_W_xu input; estimated_W_xu_fixed output
function estimated_W_xu_fixed = padVariableSize(estimated_W_xu)
    %#codegen
    % Declare fixed-size array
    estimated_W_xu_fixed = zeros(1, 7);
    
    % Fill the array with the variable-size signal
    estimated_W_xu_fixed(1:numel(estimated_W_xu)) = estimated_W_xu;
end

== matlab function PF_Simulink_TEST/Particle FIlter 1/Likelihood+Ipdate_Weights/MATLAB Function2 ==
  data: X_sim input; U_star input; likelihoods output size=[num_particles,1]; predicted input; iteration input
function likelihoods = computeLikelihood(X_sim, U_star, predicted, iteration)
    % Inputs:
    % X_sim: Actual state trajectory (Nx1)
    % U_star: Actual control inputs (Nu x 1)
    % predicted: A matrix containing both predicted trajectory and control inputs (14 x num_particles)
    % iteration: Current iteration index from the for iterator
%     likelihoods = zeros(num_particles,1);

    % Persistent variable to store likelihoods
    persistent likelihood_storage;

    if isempty(likelihood_storage) % Initialize on the first call
        likelihood_storage = []; % Initialize as an empty array
    end

    % Parameters
    std_state = [0.1; 0.1; 0.01; 0.05; 0.02];  % For (x, y, theta, velocity, steering)
    std_control = [0.1; 0.01];  % For (acceleration, steering rate)

    % Extract predicted trajectory and control inputs for the current particle
    predicted_trajectory = predicted(1:10, 1); % First 10 elements for states
    predicted_control = predicted(11:14, 1);   % Last 4 elements for control inputs

    % Compute the deviation between predicted and observed state trajectory
    state_deviation = X_sim - predicted_trajectory;

    % Compute the deviation between predicted and observed control inputs
    control_deviation = U_star - predicted_control;

    % Compute weighted errors
    weighted_state_error = sum(state_deviation.^2);
    weighted_control_error = sum(control_deviation.^2);

    % Combine state and control errors
    total_error = weighted_state_error + weighted_control_error;
    scaling_factor = 10 / (max(std(state_deviation(:)), std(control_deviation(:))) + 1e-5); % Adjust as necessary

    % Compute likelihood
    likelihood = exp(-0.5 * scaling_factor * total_error);
    likelihood = max(likelihood, 1e-30); % Ensure likelihood is within reasonable range

    % Store the likelihood
    likelihood_storage = [likelihood_storage; likelihood]; % Append to storage

    % Output the accumulated likelihoods
    likelihoods = likelihood_storage; % Output the accumulated likelihoods
end

== matlab function PF_Simulink_TEST/Particle Filter 2/Likelihood+Ipdate_Weights1/MATLAB Function ==
  data: X_sim2 input; U_star2 input; likelihoods2 output size=[num_particles,1]; predicted2 input; iteration2 input; num_particles2 input
function likelihoods2 = computeLikelihood1(X_sim2, U_star2, predicted2, iteration2, num_particles2)
    % Inputs:
    % X_sim: Actual state trajectory (Nx1)
    % U_star: Actual control inputs (Nu x 1)
    % predicted: A matrix containing both predicted trajectory and control inputs (14 x num_particles)
    % iteration: Current iteration index from the for iterator
    % num_particles: Number of particles used

%     % Initialize likelihood_storage to zeros at the start of each PF
%     persistent likelihood_storage;
% 
%     % Initialize on the first call or reset after each PF
%     if isempty(likelihood_storage) || length(likelihood_storage) ~= num_particles
%         likelihood_storage = zeros(num_particles, 1); % Initialize as zeros
%     end
    likelihood_storage=zeros(num_particles2,1);

    % Parameters
    std_state = [0.1; 0.1; 0.01; 0.05; 0.02];  % For (x, y, theta, velocity, steering)
    std_control = [0.1; 0.01];  % For (acceleration, steering rate)

    % Extract predicted trajectory and control inputs for the current particle
%     predicted_trajectory = predicted2(1:10); % First 10 elements for states
%     predicted_control = predicted2(11:14);   % Last 4 elements for control inputs
    predicted_trajectory = predicted2(1:5); % First 10 elements for states
    predicted_control = predicted2(11:12);   % Last 4 elements for control inputs
    % Compute the deviation between predicted and observed state trajectory
    state_deviation = X_sim2 - predicted_trajectory;

    % Compute the deviation between predicted and observed control inputs
    control_deviation = U_star2 - predicted_control;

    % Compute weighted errors
    weighted_state_error = sum(state_deviation.^2);
    weighted_control_error = sum(control_deviation.^2);

    % Combine state and control errors
    total_error = weighted_state_error + weighted_control_error;
    scaling_factor = 10 / (max(std(state_deviation(:)), std(control_deviation(:))) + 1e-5); % Adjust as necessary

    % Compute likelihood
    likelihood = exp(-0.5 * scaling_factor * total_error);
    likelihood = max(likelihood, 1e-30); % Ensure likelihood is within reasonable range

    % Update the likelihood storage for the current iteration
    likelihood_storage(iteration2) = likelihood;

    % Output the accumulated likelihoods
    likelihoods2 = likelihood_storage; % Output the accumulated likelihoods
end

== matlab function PF_Simulink_TEST/MATLAB Function1 ==
  data: lbu output
function lbu = LBU
% Define lower bounds for control inputs
lbu_control = [-11.5; -1; -11.5; -1]; % Control inputs

% Determine how many times to repeat the control bounds
num_repeats = ceil(80 / length(lbu_control)); % Calculate how many times to repeat
lbu = repmat(lbu_control, num_repeats, 1); % Repeat to create a long enough array
lbu = lbu(1:80); % Truncate to exactly 80 elements

% Check size
assert(length(lbu) == 80, 'Lower bounds array must have 80 elements.');

end

== matlab function PF_Simulink_TEST/Particle Filter 2/Likelihood+Ipdate_Weights1/MATLAB Function1 ==
  data: X_sim input; U_star input; likelihoods output; predicted input
% function [likelihood, total_error] = computeLikelihood(X_sim, predicted_trajectory, U_star)
%     % Extract state and control inputs
%     nx = 10;  % Number of state variables
%     nu = 4;   % Number of control inputs
% 
%     % Assuming predicted_trajectory is a 14x1 vector
%     predicted_states = predicted_trajectory(1:nx); % First 10 elements for states
%     predicted_control = predicted_trajectory(nx+1:end); % Last 4 elements for controls
% 
%     std_state = [0.1; 0.1; 0.01; 0.05; 0.02];  % For (x, y, theta, velocity, steering)
%     std_control = [0.1; 0.01];  % For (acceleration, steering rate)
% 
%     % Compute the deviation between predicted and observed state trajectory
%     state_deviation = X_sim - predicted_states;
% 
%     % Compute the deviation between predicted and observed control inputs
%     control_deviation = U_star - predicted_control;
% 
%     % Assuming state variables are weighted
%     importance_state_weights = [1, 1, 1e-5, 1e-5, 1e-5]; % Weights for state variables
%     importance_control_weights = [1, 1];                 % Weights for control inputs
%     
%     % Noise-based weights
%     noise_state_weights = 1 ./ (2 * std_state.^2);  % State noise
%     noise_control_weights = 2 * std_control.^2;  % Control noise
% 
%     combined_state_weights = importance_state_weights ./ (1 + noise_state_weights);
%     normalized_weights_state = combined_state_weights / sum(combined_state_weights);
% 
%     combined_control_weights = importance_control_weights .* (1 ./ (1 + noise_control_weights));
%     normalized_weights_control = combined_control_weights / sum(combined_control_weights);
% 
%     % Compute weighted state and control errors
%     weighted_state_error = sum((normalized_weights_state' .* state_deviation).^2, 1);
%     weighted_control_error = sum((normalized_weights_control' .* control_deviation).^2, 1);
% 
%     % Combine state and control errors
%     total_error = sum(weighted_state_error) + sum(weighted_control_error);
% 
%     norm_state_error = state_deviation ./ (std(state_deviation(:)) + 1e-5);
%     norm_control_error = control_deviation ./ (std(control_deviation(:)) + 1e-5);
%     
%     scaling_factor = 10 * 1 / (max(std(norm_state_error), std(norm_control_error)) + 1e-5);
% 
%     % Compute likelihood
%     likelihood = exp(-0.5 * scaling_factor * total_error);
%     likelihood = max(likelihood, 1e-30); % Ensure likelihood is within a reasonable range
% end

function likelihoods = computeLikelihoods(X_sim, U_star, predicted)
    % Inputs:
    % X_sim: Actual state trajectory (Nx1)
    % U_star: Actual control inputs (Nu x 1)
    % predicted: A matrix containing both predicted trajectory and control inputs (14 x num_particles)

    % Parameters
    num_particles = size(predicted, 2); % Number of particles
    likelihoods = zeros(num_particles, 1); % Preallocate array for likelihoods

    std_state = [0.1; 0.1; 0.01; 0.05; 0.02];  % For (x, y, theta, velocity, steering)
    std_control = [0.1; 0.01];  % For (acceleration, steering rate)

    % Loop through each particle
    for i = 1:num_particles
        % Extract predicted trajectory and control inputs for the current particle
        predicted_trajectory = predicted(1:10, i); % First 10 elements for states
        predicted_control = predicted(11:14, i);   % Last 4 elements for control inputs

        % Compute the deviation between predicted and observed state trajectory
        state_deviation = X_sim - predicted_trajectory;

        % Compute the deviation between predicted and observed control inputs
        control_deviation = U_star - predicted_control;

        % Compute weighted errors (adjust according to your weighting scheme)
        weighted_state_error = sum(state_deviation.^2);
        weighted_control_error = sum(control_deviation.^2);

        % Combine state and control errors
        total_error = weighted_state_error + weighted_control_error;
        scaling_factor = 10 / (max(std(state_deviation(:)), std(control_deviation(:))) + 1e-5); % Adjust as necessary

        % Compute likelihood
        likelihood = exp(-0.5 * scaling_factor * total_error);
        likelihood = max(likelihood, 1e-30); % Ensure likelihood is within reasonable range

        % Store the likelihood for this particle
        likelihoods(i) = likelihood;
    end
end

== matlab function PF_Simulink_TEST/Particle Filter 2/MATLAB Function6 ==
  data: W_xu2 input; W_xu2 output; resampled_weights2 output size=[num_particles,1]; weights2 input; num_particles2 input; estimated_W_xu2 output size=[1,7]; range_factor1 input; range_factor1 output
function [W_xu2, resampled_weights2,estimated_W_xu2,range_factor1] = resampleParticles1(W_xu2, weights2,num_particles2,range_factor1)
    % Inputs:
    % - W_xu: Matrix of particle states and weights (num_particles x 7)
    % - weights: Current particle weights (num_particles x 1)
    %
    % Outputs:
    % - W_xu: Resampled particle matrix (num_particles x 7)
    % - resampled_weights: Uniform weights after resampling (num_particles x 1)

  
    % Normalize weights
%     weights = weights / sum(weights);

    % Resample particle indices based on the updated weights
    estimated_W_xu2=zeros(1,7);
    resampled_weights2=zeros(num_particles2,1);

    resample_indices = randsample(1:num_particles2, num_particles2, true, weights2);

    % Resample particles using the indices
    W_xu2 = W_xu2(resample_indices, :); 

    % Reset weights to uniform distribution after resampling
    resampled_weights2 = ones(num_particles2, 1) / num_particles2;

    % Return the updated W_xu, pre-resample weights, and resampled weights


     % Element-wise multiplication of W_xu by weights
    weighted_W_xu = W_xu2 .* resampled_weights2;

    % Sum the weighted values across the particles (i.e., summing along rows)
    estimated_W_xu2 = sum(weighted_W_xu, 1); % Output will be 1x7
    range_factor1=range_factor1*0.9975;
    range_factor1=max(0.10,range_factor1);
end

== matlab function PF_Simulink_TEST/Particle Filter 2/MATLAB Function9 ==
  data: estimated_W_xu2 input; estimated_W_xu_fixed2 output
function estimated_W_xu_fixed2 = padVariableSize1(estimated_W_xu2)
    %#codegen
    % Declare fixed-size array
    estimated_W_xu_fixed2 = zeros(1, 7);
    
    % Fill the array with the variable-size signal
    estimated_W_xu_fixed2(1:numel(estimated_W_xu2)) = estimated_W_xu2;
end

== matlab function PF_Simulink_TEST/Particle Filter 2/PF_pred_trajectories2/MATLAB Function ==
  data: u1 input; Y1 output size=[14,num_particles]; i1 input
function Y1 = fcn1(u1, i1)
    persistent Y_storage; % Declare Y_storage as a persistent variable

    if isempty(Y_storage) % Initialize on the first call
        Y_storage = []; % Initialize as an empty array
    end

    if i1 == 1
        Y_storage = u1; % Assign the first input directly
    else
        Y_storage = [Y_storage u1]; % Concatenate the new input
    end

    Y1 = Y_storage; % Output the accumulated results
end
